simulink model "my_robot_2"  (R2013a)
settings: Solver=ode4  StartTime=0.0  StopTime=T  FixedStep=1/fs  RelTol=1e-3
values from neighbouring files (symbols this model uses):
  Kp = eye(robot.n) * k * (pi*fs)^2    [Ejercicio1.m]    (also in Ejercicio2.m = Kp/Wall.Ke)
  Kv = 2*sqrt(Kp)    [Ejercicio1.m]    (also in Ejercicio2.m)
  thetai = robot.ikine(Ti, [0, pi/2], [1 1 0 0 0 0])    [Ejercicio1.m]    (also in Ejercicio2.m; Ejercicio3.m)
settings Model: Creator=Juan Pablo  LastModifiedBy=root
settings DataIOCC: ExternalInput=[t, FSetpoint]  LimitDataPoints=off  LoadExternalInput=on  SaveTime=off  OutputSaveName=q, x, Fe, F, tau

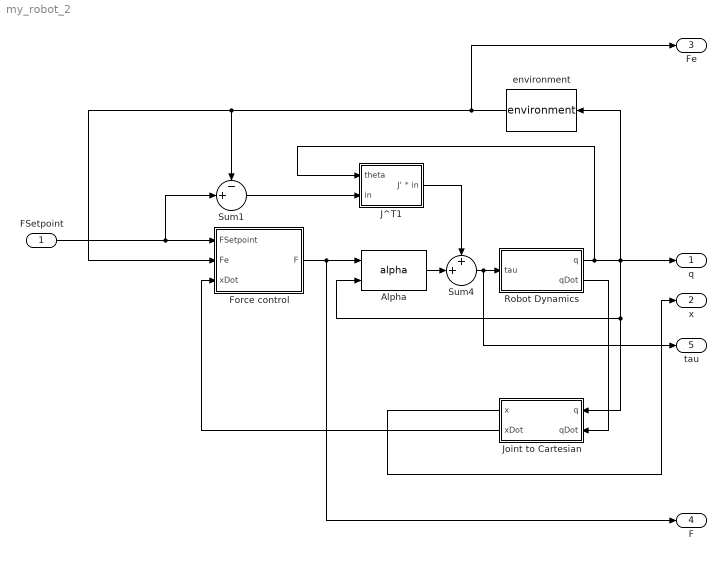
== system my_robot_2 ==
  FSetpoint : Inport  PortDimensions=2
  Alpha : M-S-Function  FunctionName=alpha  Parameters=robot
  Force control : Subsystem
  J^T1 : Subsystem
  Joint to Cartesian : Subsystem
  Robot Dynamics : Subsystem
  Sum1 : Sum  Inputs=-+|
  Sum4 : Sum  Inputs=++|
  environment : M-S-Function  FunctionName=environment  Parameters=robot, Wall
  q : Outport
  x : Outport  Port=2
  Fe : Outport  Port=3
  F : Outport  Port=4
  tau : Outport  Port=5
  wires:
  Robot Dynamics/1(q) -> J^T1/1(theta), environment/1, q/1, Alpha/2, Joint to Cartesian/1(q)
  Robot Dynamics/2(qDot) -> Joint to Cartesian/2(qDot)
  Joint to Cartesian/1(x) -> x/1
  Sum4/1 -> tau/1, Robot Dynamics/1(tau)
  FSetpoint/1 -> Sum1/2, Force control/1(FSetpoint)
  Joint to Cartesian/2(xDot) -> Force control/3(xDot)
  environment/1 -> Fe/1, Sum1/1, Force control/2(Fe)
  Force control/1(F) -> F/1, Alpha/1
  Alpha/1 -> Sum4/2
  J^T1/1(J' * in) -> Sum4/1
  Sum1/1 -> J^T1/2(in)

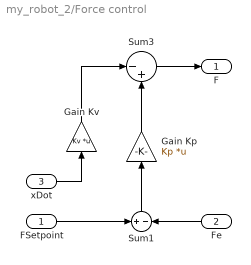
== system my_robot_2/Force control ==
  FSetpoint : Inport
  Fe : Inport  Port=2
  xDot : Inport  Port=3
  Gain Kp : Gain  Gain=Kp  Multiplication=Matrix(K*u)
  Gain Kv : Gain  Gain=Kv  Multiplication=Matrix(K*u)
  Sum1 : Sum  Inputs=+|-
  Sum3 : Sum  Inputs=|-+
  F : Outport
  wires:
  Fe/1 -> Sum1/2
  FSetpoint/1 -> Sum1/1
  Sum1/1 -> Gain Kp/1
  Sum3/1 -> F/1
  Gain Kp/1 -> Sum3/2
  xDot/1 -> Gain Kv/1
  Gain Kv/1 -> Sum3/1

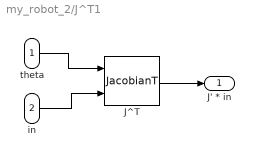
== system my_robot_2/J^T1 ==
  theta : Inport
  in : Inport  Port=2
  J^T : M-S-Function  FunctionName=JacobianT  Parameters=robot
  J' * in : Outport
  wires:
  theta/1 -> J^T/1
  J^T/1 -> J' * in/1
  in/1 -> J^T/2

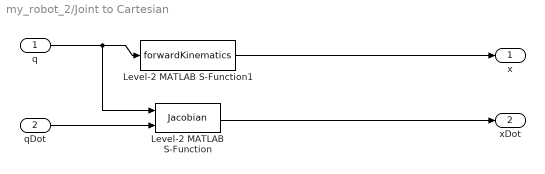
== system my_robot_2/Joint to Cartesian ==
  q : Inport
  qDot : Inport  Port=2
  Level-2 MATLAB S-Function : M-S-Function  FunctionName=Jacobian  Parameters=robot
  Level-2 MATLAB S-Function1 : M-S-Function  FunctionName=forwardKinematics  Parameters=robot
  x : Outport
  xDot : Outport  Port=2
  wires:
  q/1 -> Level-2 MATLAB S-Function1/1, Level-2 MATLAB S-Function/1
  qDot/1 -> Level-2 MATLAB S-Function/2
  Level-2 MATLAB S-Function/1 -> xDot/1
  Level-2 MATLAB S-Function1/1 -> x/1

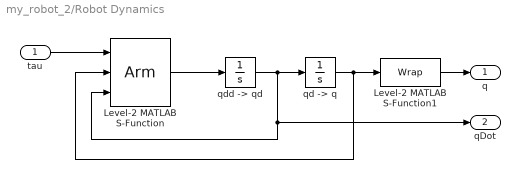
== system my_robot_2/Robot Dynamics ==
  tau : Inport
  Level-2 MATLAB S-Function : M-S-Function  FunctionName=Arm  Parameters=probot
  Level-2 MATLAB S-Function1 : M-S-Function  FunctionName=Wrap  Parameters=robot
  "qd -> q" : Integrator  InitialCondition=thetai
  "qdd -> qd" : Integrator
  q : Outport
  qDot : Outport  Port=2
  wires:
  Level-2 MATLAB S-Function/1 -> "qdd -> qd"/1
  "qdd -> qd"/1 -> Level-2 MATLAB S-Function/3, qDot/1, "qd -> q"/1
  "qd -> q"/1 -> Level-2 MATLAB S-Function/2, Level-2 MATLAB S-Function1/1
  tau/1 -> Level-2 MATLAB S-Function/1
  Level-2 MATLAB S-Function1/1 -> q/1
